simulink model "myStateFlow"  (R2018b)
settings: Solver=FixedStepAuto  StartTime=0.0  StopTime=2555  FixedStep=Ts  RelTol=1e-3
undefined symbols (not defined in the file or in its folder): DiscIntNeverNeededParam, plannedpath, pos0, posf
libraries: simulink x3
(part 1 of 2)
settings Model: Creator=sl  LastModifiedBy=sl

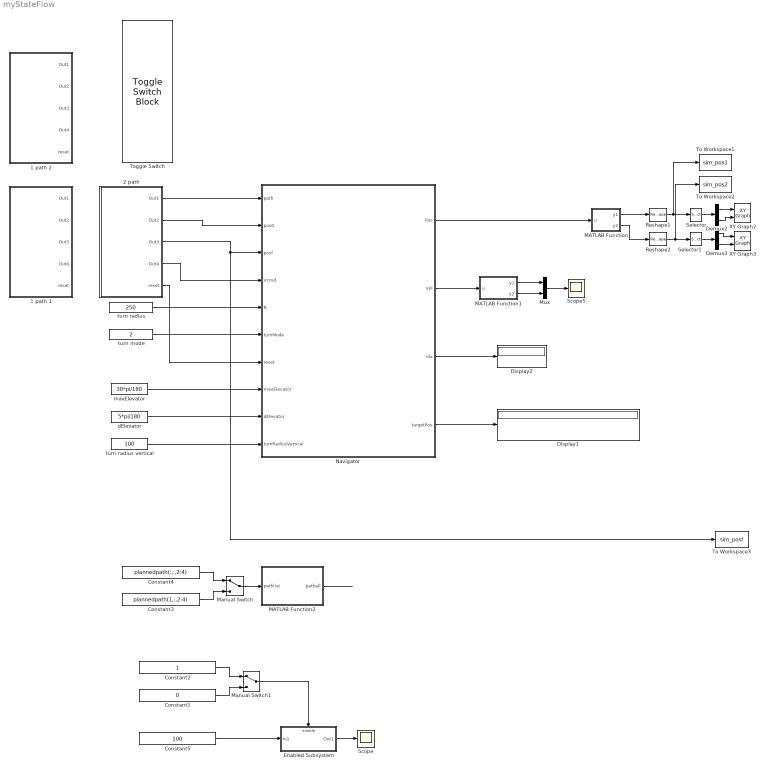
== system myStateFlow ==
  1 path 1 : Subsystem
  1 path 2 : Subsystem
  2 path : Subsystem
  Constant1 : Constant  Value=0  VectorParams1D=off
  Constant2 : Constant  VectorParams1D=off
  Constant3 : Constant  Value=plannedpath(1,:,2:4)  VectorParams1D=off
  Constant4 : Constant  Value=plannedpath(:,:,2:4)  VectorParams1D=off
  Constant5 : Constant  Value=100  VectorParams1D=off
  Demux2 : Demux  Outputs=2
  Demux3 : Demux  Outputs=2
  Display1 : Display
  Display2 : Display
  Enabled Subsystem : Subsystem  TreatAsAtomicUnit=on
  MATLAB Function : MATLAB Function  TreatAsAtomicUnit=on
  MATLAB Function1 : MATLAB Function  TreatAsAtomicUnit=on
  MATLAB Function2 : MATLAB Function  TreatAsAtomicUnit=on
  Manual Switch : ManualSwitch  varsize=on
  Manual Switch1 : ManualSwitch
  Mux : Mux  Inputs=2
  Navigator : Subsystem
  Reshape1 : Reshape
  Reshape2 : Reshape
  Scope : Scope
  Scope5 : Scope
  Selector : Selector  InputPortWidth=3  IndexOptions=Index vector (dialog)  Indices=[1 2]  OutputSizes=1
  Selector1 : Selector  InputPortWidth=3  IndexOptions=Index vector (dialog)  Indices=[1 2]  OutputSizes=1
  To Workspace1 : ToWorkspace  VariableName=sim_pos1  SaveFormat=Timeseries  SampleTime=-1
  To Workspace2 : ToWorkspace  VariableName=sim_pos2  SaveFormat=Timeseries  SampleTime=-1
  To Workspace3 : ToWorkspace  VariableName=sim_posf  SaveFormat=Timeseries  SampleTime=-1
  Toggle Switch : ToggleSwitchBlock  Tag=Reset  WebBlockId=267
      settings: Values={{'Off', 'On'}, [0 1]}
  XY Graph2 : simulink/Sinks/XY Graph  xmin=-2e4  xmax=2e4  ymin=-2e4  ymax=2e4  st=-1
  XY Graph3 : simulink/Sinks/XY Graph  xmin=-2e4  xmax=2e4  ymin=-2e4  ymax=2e4  st=-1
  dElevator : Constant  Value=5*pi/180
  maxElevator : Constant  Value=30*pi/180
  turn mode : Constant  Value=2  VectorParams1D=off
  turn radius : Constant  Value=250  VectorParams1D=off
  turn radius vertical : Constant  Value=100
  wires:
  Navigator/1(Pos) -> MATLAB Function/1(u)
  MATLAB Function/1(y1) -> Reshape1/1
  MATLAB Function/2(y2) -> Reshape2/1
  Demux2/1 -> XY Graph2/1
  Demux2/2 -> XY Graph2/2
  Demux3/2 -> XY Graph3/2
  Demux3/1 -> XY Graph3/1
  Reshape2/1 -> Selector1/1, To Workspace2/1
  Reshape1/1 -> To Workspace1/1, Selector/1
  Selector/1 -> Demux2/1
  Selector1/1 -> Demux3/1
  Navigator/2(Vel) -> MATLAB Function1/1(u)
  MATLAB Function1/1(y1) -> Mux/1
  MATLAB Function1/2(y2) -> Mux/2
  Mux/1 -> Scope5/1
  Navigator/3(idx) -> Display2/1
  Constant4/1 -> Manual Switch/1
  Constant3/1 -> Manual Switch/2
  Manual Switch/1 -> MATLAB Function2/1(pathlist)
  MATLAB Function2/1(pathall) -> ?
  2 path/3(Out3) -> Navigator/3(posf), To Workspace3/1
  2 path/1(Out1) -> Navigator/1(path)
  2 path/2(Out2) -> Navigator/2(pos0)
  2 path/4(Out4) -> Navigator/4(Vcmd)
  turn radius/1 -> Navigator/5(R)
  turn mode/1 -> Navigator/6(turnMode)
  maxElevator/1 -> Navigator/8(maxElevator)
  dElevator/1 -> Navigator/9(dElevator)
  turn radius vertical/1 -> Navigator/10("turnRadiusVertical ")
  Navigator/4(targetPos) -> Display1/1
  2 path/5(reset) -> Navigator/7(reset)
  Constant1/1 -> Manual Switch1/2
  Constant2/1 -> Manual Switch1/1
  Manual Switch1/1 -> Enabled Subsystem/Enable
  Constant5/1 -> Enabled Subsystem/1(In1)
  Enabled Subsystem/1(Out1) -> Scope/1

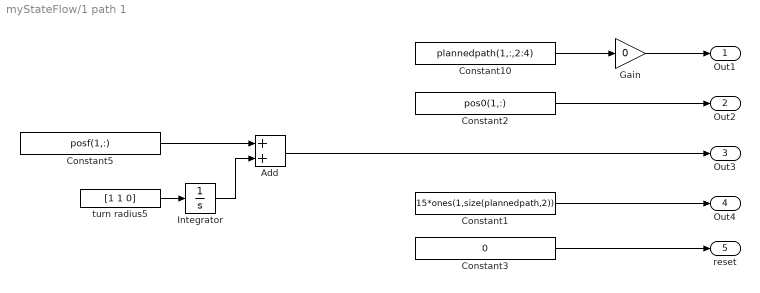
== system myStateFlow/1 path 1 ==
  Add : Sum
  Constant1 : Constant  Value=15*ones(1,size(plannedpath,2))  VectorParams1D=off
  Constant10 : Constant  Value=plannedpath(1,:,2:4)  VectorParams1D=off
  Constant2 : Constant  Value=pos0(1,:)  VectorParams1D=off
  Constant3 : Constant  Value=0  VectorParams1D=off
  Constant5 : Constant  Value=posf(1,:)  VectorParams1D=off
  Gain : Gain  Gain=0
  Integrator : Integrator
  turn radius5 : Constant  Value=[1 1 0]  VectorParams1D=off
  Out1 : Outport
  Out2 : Outport  Port=2
  Out3 : Outport  Port=3
  Out4 : Outport  Port=4
  reset : Outport  Port=5
  wires:
  Constant5/1 -> Add/1
  Add/1 -> Out3/1
  Integrator/1 -> Add/2
  Constant1/1 -> Out4/1
  turn radius5/1 -> Integrator/1
  Constant10/1 -> Gain/1
  Constant2/1 -> Out2/1
  Gain/1 -> Out1/1
  Constant3/1 -> reset/1

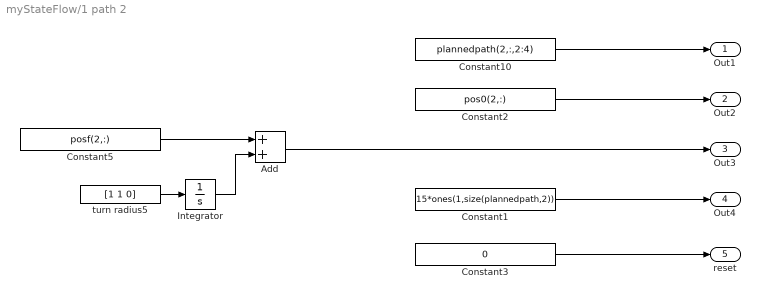
== system myStateFlow/1 path 2 ==
  Add : Sum
  Constant1 : Constant  Value=15*ones(1,size(plannedpath,2))  VectorParams1D=off
  Constant10 : Constant  Value=plannedpath(2,:,2:4)  VectorParams1D=off
  Constant2 : Constant  Value=pos0(2,:)  VectorParams1D=off
  Constant3 : Constant  Value=0  VectorParams1D=off
  Constant5 : Constant  Value=posf(2,:)  VectorParams1D=off
  Integrator : Integrator
  turn radius5 : Constant  Value=[1 1 0]  VectorParams1D=off
  Out1 : Outport
  Out2 : Outport  Port=2
  Out3 : Outport  Port=3
  Out4 : Outport  Port=4
  reset : Outport  Port=5
  wires:
  Constant2/1 -> Out2/1
  Constant10/1 -> Out1/1
  turn radius5/1 -> Integrator/1
  Constant1/1 -> Out4/1
  Integrator/1 -> Add/2
  Add/1 -> Out3/1
  Constant5/1 -> Add/1
  Constant3/1 -> reset/1

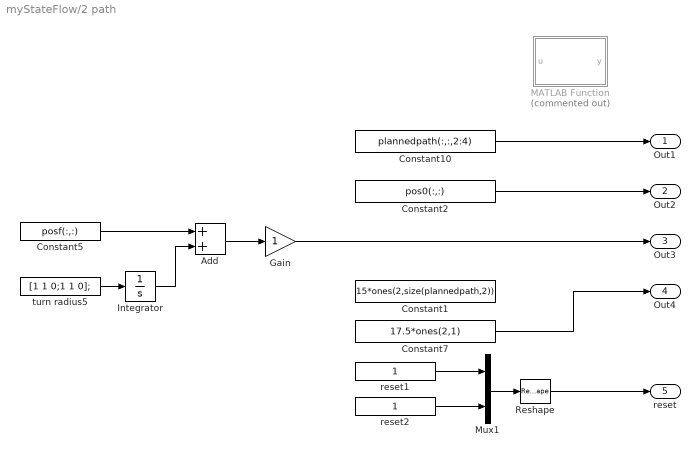
== system myStateFlow/2 path ==
  Add : Sum
  Constant1 : Constant  Value=15*ones(2,size(plannedpath,2))  VectorParams1D=off
  Constant10 : Constant  Value=plannedpath(:,:,2:4)  VectorParams1D=off
  Constant2 : Constant  Value=pos0(:,:)  VectorParams1D=off
  Constant5 : Constant  Value=posf(:,:)  VectorParams1D=off
  Constant7 : Constant  Value=17.5*ones(2,1)  VectorParams1D=off
  Gain : Gain
  Integrator : Integrator
  MATLAB Function : MATLAB Function  Commented=on  TreatAsAtomicUnit=on
  Mux1 : Mux  Inputs=2
  Reshape : Reshape  OutputDimensionality=Column vector (2-D)
  reset1 : Constant  VectorParams1D=off
  reset2 : Constant  VectorParams1D=off
  turn radius5 : Constant  Value=[1 1 0;1 1 0];  VectorParams1D=off
  Out1 : Outport
  Out2 : Outport  Port=2
  Out3 : Outport  Port=3
  Out4 : Outport  Port=4
  reset : Outport  Port=5
  wires:
  Constant2/1 -> Out2/1
  turn radius5/1 -> Integrator/1
  Integrator/1 -> Add/2
  Add/1 -> Gain/1
  Constant5/1 -> Add/1
  Constant7/1 -> Out4/1
  Gain/1 -> Out3/1
  Constant10/1 -> Out1/1
  Reshape/1 -> reset/1
  Mux1/1 -> Reshape/1
  reset1/1 -> Mux1/1
  reset2/1 -> Mux1/2

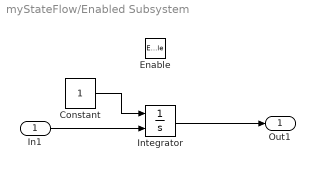
== system myStateFlow/Enabled Subsystem ==
  In1 : Inport
  Enable : EnablePort
  Constant : Constant
  Integrator : Integrator  InitialConditionSource=external
  Out1 : Outport
  wires:
  In1/1 -> Integrator/2
  Integrator/1 -> Out1/1
  Constant/1 -> Integrator/1

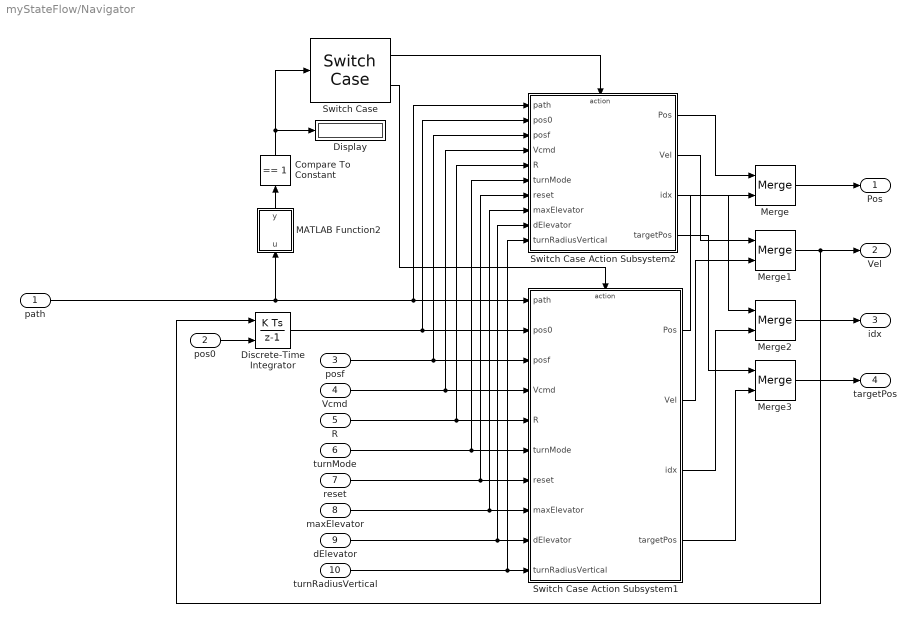
== system myStateFlow/Navigator ==
  path : Inport
  pos0 : Inport  Port=2
  posf : Inport  Port=3
  Vcmd : Inport  Port=4
  R : Inport  Port=5
  turnMode : Inport  Port=6
  reset : Inport  Port=7
  maxElevator : Inport  Port=8
  dElevator : Inport  Port=9
  "turnRadiusVertical " : Inport  Port=10
  Compare To Constant : simulink/Logic and Bit Operations/Compare To Constant  relop===  const=1  OutDataTypeStr=uint8
  Discrete-Time Integrator : DiscreteIntegrator  InitialConditionSource=external  SampleTime=-1  ICPrevOutput=DiscIntNeverNeededParam  ICPrevScaledInput=DiscIntNeverNeededParam
  Display : Display
  MATLAB Function2 : MATLAB Function  TreatAsAtomicUnit=on
  Merge{,1..3} (4 alike) : Merge
  Switch Case : SwitchCase
  Switch Case Action Subsystem1 : Subsystem  TreatAsAtomicUnit=on
  Switch Case Action Subsystem2 : Subsystem  TreatAsAtomicUnit=on
  Pos : Outport
  Vel : Outport  Port=2
  idx : Outport  Port=3
  targetPos : Outport  Port=4
  wires:
  pos0/1 -> Discrete-Time Integrator/2
  Switch Case Action Subsystem2/4(targetPos) -> Merge3/1
  Switch Case Action Subsystem1/4(targetPos) -> Merge3/2
  Merge3/1 -> targetPos/1
  "turnRadiusVertical "/1 -> Switch Case Action Subsystem1/10("turnRadiusVertical "), Switch Case Action Subsystem2/10("turnRadiusVertical ")
  dElevator/1 -> Switch Case Action Subsystem1/9(dElevator), Switch Case Action Subsystem2/9(dElevator)
  maxElevator/1 -> Switch Case Action Subsystem1/8(maxElevator), Switch Case Action Subsystem2/8(maxElevator)
  path/1 -> MATLAB Function2/1(u), Switch Case Action Subsystem1/1(path), Switch Case Action Subsystem2/1(path)
  reset/1 -> Switch Case Action Subsystem1/7(reset), Switch Case Action Subsystem2/7(reset)
  turnMode/1 -> Switch Case Action Subsystem1/6(turnMode), Switch Case Action Subsystem2/6(turnMode)
  Switch Case Action Subsystem2/2(Vel) -> Merge1/1
  Switch Case Action Subsystem2/1(Pos) -> Merge/1
  Switch Case Action Subsystem1/2(Vel) -> Merge1/2
  Switch Case Action Subsystem2/3(idx) -> Merge2/1
  Switch Case/2 -> Switch Case Action Subsystem1/Action
  Switch Case/1 -> Switch Case Action Subsystem2/Action
  posf/1 -> Switch Case Action Subsystem1/3(posf), Switch Case Action Subsystem2/3(posf)
  Merge1/1 -> Vel/1, Discrete-Time Integrator/1
  Merge2/1 -> idx/1
  Vcmd/1 -> Switch Case Action Subsystem1/4(Vcmd), Switch Case Action Subsystem2/4(Vcmd)
  MATLAB Function2/1(y) -> Compare To Constant/1
  R/1 -> Switch Case Action Subsystem1/5(R), Switch Case Action Subsystem2/5(R)
  Compare To Constant/1 -> Switch Case/1, Display/1
  Discrete-Time Integrator/1 -> Switch Case Action Subsystem1/2(pos0), Switch Case Action Subsystem2/2(pos0)
  Switch Case Action Subsystem1/3(idx) -> Merge2/2
  Switch Case Action Subsystem1/1(Pos) -> Merge/2
  Merge/1 -> Pos/1

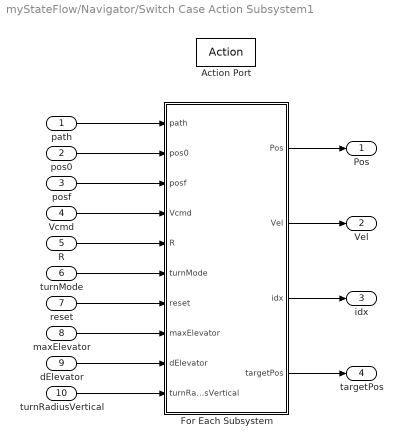
== system myStateFlow/Navigator/Switch Case Action Subsystem1 ==
  path : Inport
  pos0 : Inport  Port=2
  posf : Inport  Port=3
  Vcmd : Inport  Port=4
  R : Inport  Port=5
  turnMode : Inport  Port=6
  reset : Inport  Port=7
  maxElevator : Inport  Port=8
  dElevator : Inport  Port=9
  "turnRadiusVertical " : Inport  Port=10
  Action Port : ActionPort
  For Each Subsystem : Subsystem  TreatAsAtomicUnit=on
  Pos : Outport
  Vel : Outport  Port=2
  idx : Outport  Port=3
  targetPos : Outport  Port=4
  wires:
  For Each Subsystem/4(targetPos) -> targetPos/1
  "turnRadiusVertical "/1 -> For Each Subsystem/10("turnRadiusVertical ")
  dElevator/1 -> For Each Subsystem/9(dElevator)
  maxElevator/1 -> For Each Subsystem/8(maxElevator)
  reset/1 -> For Each Subsystem/7(reset)
  turnMode/1 -> For Each Subsystem/6(turnMode)
  path/1 -> For Each Subsystem/1(path)
  pos0/1 -> For Each Subsystem/2(pos0)
  posf/1 -> For Each Subsystem/3(posf)
  Vcmd/1 -> For Each Subsystem/4(Vcmd)
  R/1 -> For Each Subsystem/5(R)
  For Each Subsystem/1(Pos) -> Pos/1
  For Each Subsystem/2(Vel) -> Vel/1
  For Each Subsystem/3(idx) -> idx/1

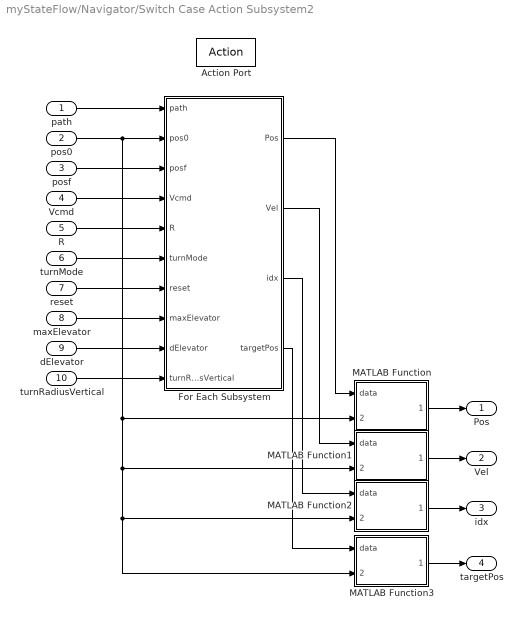
== system myStateFlow/Navigator/Switch Case Action Subsystem2 ==
  path : Inport
  pos0 : Inport  Port=2
  posf : Inport  Port=3
  Vcmd : Inport  Port=4
  R : Inport  Port=5
  turnMode : Inport  Port=6
  reset : Inport  Port=7
  maxElevator : Inport  Port=8
  dElevator : Inport  Port=9
  "turnRadiusVertical " : Inport  Port=10
  Action Port : ActionPort
  For Each Subsystem : Subsystem  TreatAsAtomicUnit=on
  MATLAB Function : MATLAB Function  TreatAsAtomicUnit=on
  MATLAB Function1 : MATLAB Function  TreatAsAtomicUnit=on
  MATLAB Function2 : MATLAB Function  TreatAsAtomicUnit=on
  MATLAB Function3 : MATLAB Function  TreatAsAtomicUnit=on
  Pos : Outport
  Vel : Outport  Port=2
  idx : Outport  Port=3
  targetPos : Outport  Port=4
  wires:
  MATLAB Function3/1(dataout) -> targetPos/1
  For Each Subsystem/4(targetPos) -> MATLAB Function3/1(data)
  "turnRadiusVertical "/1 -> For Each Subsystem/10("turnRadiusVertical ")
  dElevator/1 -> For Each Subsystem/9(dElevator)
  maxElevator/1 -> For Each Subsystem/8(maxElevator)
  reset/1 -> For Each Subsystem/7(reset)
  turnMode/1 -> For Each Subsystem/6(turnMode)
  MATLAB Function2/1(dataout) -> idx/1
  MATLAB Function1/1(dataout) -> Vel/1
  MATLAB Function/1(dataout) -> Pos/1
  For Each Subsystem/3(idx) -> MATLAB Function2/1(data)
  For Each Subsystem/2(Vel) -> MATLAB Function1/1(data)
  For Each Subsystem/1(Pos) -> MATLAB Function/1(data)
  R/1 -> For Each Subsystem/5(R)
  Vcmd/1 -> For Each Subsystem/4(Vcmd)
  posf/1 -> For Each Subsystem/3(posf)
  pos0/1 -> For Each Subsystem/2(pos0), MATLAB Function1/2(sizedata), MATLAB Function2/2(sizedata), MATLAB Function3/2(sizedata), MATLAB Function/2(sizedata)
  path/1 -> For Each Subsystem/1(path)

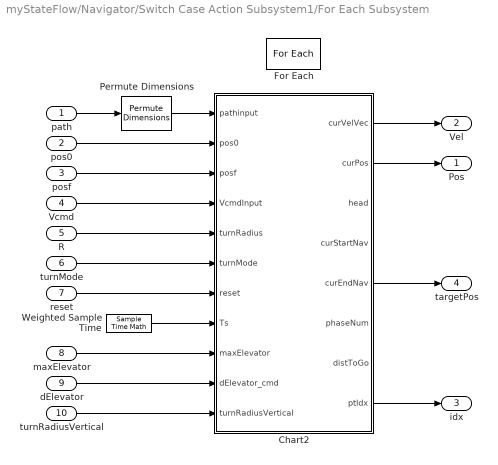
== system myStateFlow/Navigator/Switch Case Action Subsystem1/For Each Subsystem ==
  path : Inport  Partition=on  PartitionDimension=1  PartitionWidth=1  PartitionOffset=0
  pos0 : Inport  Port=2  Partition=on  PartitionDimension=1  PartitionWidth=1  PartitionOffset=0
  posf : Inport  Port=3  Partition=on  PartitionDimension=1  PartitionWidth=1  PartitionOffset=0
  Vcmd : Inport  Port=4  Partition=on  PartitionDimension=1  PartitionWidth=1  PartitionOffset=0
  R : Inport  Port=5
  turnMode : Inport  Port=6
  reset : Inport  Port=7  Partition=on  PartitionDimension=1  PartitionWidth=1  PartitionOffset=0
  maxElevator : Inport  Port=8
  dElevator : Inport  Port=9
  "turnRadiusVertical " : Inport  Port=10
  Chart2 : Stateflow chart  TreatAsAtomicUnit=on
  For Each : ForEach  DisableCoverage=on  IndexMode=One-based
  Permute Dimensions : PermuteDimensions  Order=[2,3,1]
  Weighted Sample Time : SampleTimeMath  TsampMathOp=Ts Only
  Pos : Outport  ConcatenationDimension=1
  Vel : Outport  Port=2  ConcatenationDimension=1
  idx : Outport  Port=3  ConcatenationDimension=1
  targetPos : Outport  Port=4  ConcatenationDimension=1
  wires:
  Chart2/5(curEndNav) -> targetPos/1
  turnMode/1 -> Chart2/6(turnMode)
  Chart2/8(ptIdx) -> idx/1
  "turnRadiusVertical "/1 -> Chart2/11(turnRadiusVertical)
  dElevator/1 -> Chart2/10(dElevator_cmd)
  maxElevator/1 -> Chart2/9(maxElevator)
  Weighted Sample Time/1 -> Chart2/8(Ts)
  reset/1 -> Chart2/7(reset)
  Chart2/2(curPos) -> Pos/1
  R/1 -> Chart2/5(turnRadius)
  Chart2/1(curVelVec) -> Vel/1
  Vcmd/1 -> Chart2/4(VcmdInput)
  pos0/1 -> Chart2/2(pos0)
  posf/1 -> Chart2/3(posf)
  path/1 -> Permute Dimensions/1
  Permute Dimensions/1 -> Chart2/1(pathinput)

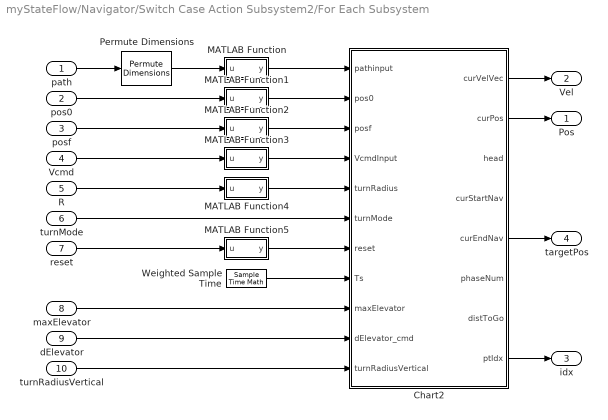
== system myStateFlow/Navigator/Switch Case Action Subsystem2/For Each Subsystem ==
  path : Inport
  pos0 : Inport  Port=2
  posf : Inport  Port=3
  Vcmd : Inport  Port=4
  R : Inport  Port=5
  turnMode : Inport  Port=6
  reset : Inport  Port=7
  maxElevator : Inport  Port=8
  dElevator : Inport  Port=9
  "turnRadiusVertical " : Inport  Port=10
  Chart2 : Stateflow chart  TreatAsAtomicUnit=on
  MATLAB Function : MATLAB Function  TreatAsAtomicUnit=on
  MATLAB Function1 : MATLAB Function  TreatAsAtomicUnit=on
  MATLAB Function2 : MATLAB Function  TreatAsAtomicUnit=on
  MATLAB Function3 : MATLAB Function  TreatAsAtomicUnit=on
  MATLAB Function4 : MATLAB Function  TreatAsAtomicUnit=on
  MATLAB Function5 : MATLAB Function  TreatAsAtomicUnit=on
  Permute Dimensions : PermuteDimensions  Order=[2,3,1]
  Weighted Sample Time : SampleTimeMath  TsampMathOp=Ts Only
  Pos : Outport
  Vel : Outport  Port=2
  idx : Outport  Port=3
  targetPos : Outport  Port=4
  wires:
  MATLAB Function5/1(y) -> Chart2/7(reset)
  Chart2/5(curEndNav) -> targetPos/1
  "turnRadiusVertical "/1 -> Chart2/11(turnRadiusVertical)
  dElevator/1 -> Chart2/10(dElevator_cmd)
  maxElevator/1 -> Chart2/9(maxElevator)
  reset/1 -> MATLAB Function5/1(u)
  turnMode/1 -> Chart2/6(turnMode)
  MATLAB Function4/1(y) -> Chart2/5(turnRadius)
  MATLAB Function3/1(y) -> Chart2/4(VcmdInput)
  MATLAB Function2/1(y) -> Chart2/3(posf)
  MATLAB Function1/1(y) -> Chart2/2(pos0)
  MATLAB Function/1(y) -> Chart2/1(pathinput)
  Permute Dimensions/1 -> MATLAB Function/1(u)
  path/1 -> Permute Dimensions/1
  posf/1 -> MATLAB Function2/1(u)
  pos0/1 -> MATLAB Function1/1(u)
  Vcmd/1 -> MATLAB Function3/1(u)
  Chart2/8(ptIdx) -> idx/1
  Chart2/1(curVelVec) -> Vel/1
  R/1 -> MATLAB Function4/1(u)
  Weighted Sample Time/1 -> Chart2/8(Ts)
  Chart2/2(curPos) -> Pos/1

== matlab function myStateFlow/MATLAB Function ==
  data: u input; y1 output; y2 output
function [y1,y2]= fcn(u)

y1 = u(1,:);
y2 = u(2,:);

== matlab function myStateFlow/MATLAB Function1 ==
  data: u input; y1 output; y2 output
function [y1,y2]= fcn(u)

y1 = norm(u(1,:));
y2 = norm(u(1,:));

== matlab function myStateFlow/MATLAB Function2 ==
  data: pathlist input; pathall output
function pathall = formPathList(pathlist)
% 将变长度航路转换为固定长度航路，便于后续处理
maxPathNum = 10;
maxPathPointNum = 100;
pathall = zeros(maxPathNum,maxPathPointNum,3);
[realPathNum,realPtNum,~] = size(pathlist);
if realPathNum>maxPathNum || realPtNum>maxPathPointNum
    error('The dimensions of pathlist exceed limits') ;
end
for i_path = 1:realPathNum
    pathall(i_path,1:realPtNum,:) = pathlist(i_path,:,:);
end

== matlab function myStateFlow/2 path/MATLAB Function ==
  data: u input; y output
function y = fcn(u)
u(2,:,:) = zeros(size(u(2,:,:)));
y = u;

== matlab function myStateFlow/Navigator/MATLAB Function2 ==
  data: u input; y output
function y = fcn(u)
if size(u,1) == 1
    y = 1;
else
    y = 0;
end

== stateflow chart myStateFlow/Navigator/Switch Case Action Subsystem1/For Each Subsystem/Chart2 ==
  state InitialPhase
    % turnMode 转弯模式 1折现转弯 2圆弧切线转弯
    en:
    ptIdx = 1;  % 当前阶段起始点在path点集中的序号
    % 导航点的位置向量
    [path,path_h,path_v] = calValidNavPts(pos0,pathinput,posf);
    Vcmd = [VcmdInput(1),VcmdInput];
    % 导航点的时间向量
    numPts = size(path,1);%determineNumPts; % 导航点数
    curPos = path(1,:); % 初始导航点作为当前阶段的目标
    phaseNum = 1;
    turnInPos = zeros(1,3);
    turnOutPos = zeros(1,3);
    curStartNav = zeros(1,3);
    curEndNav = zeros(1,3);
    curVelVec = zeros(1,3);
    curVel = zeros(1);
    posErr = zeros(1);
  state Hover
    en:
    head = 0;
    curPos = pos0;
    curVel = Vcmd(1);
    du:
    head = head+0.1*Ts;
    curVelVec = ([cos(head) sin(head) 0;-sin(head) cos(head) 0;0 0 1]*[curVel;0;0])';
    curPos = curPos + curVelVec*Ts;
    curStartNav = [0 0 0];
    curEndNav = [0 0 0];
    phaseNum = -1;
    distToGo = -1;
    ptIdx = -1;
  state MainLoop
    state linePhase
      % ------------------------------------------------------------------------------------------------
      en:
      while 1 % 跳过连续的重复点
      curStartNav = path(ptIdx,1:3);  % 当前导航段的起始点位置
      curEndNav = path(ptIdx+1,1:3); % 当前导航段的终点位置
      curVel = Vcmd(min(ptIdx,length(Vcmd))); % 当前导航段的速度
      if isequal(curStartNav(1:2),curEndNav(1:2)) % 判断连续的两个导航点是否重合
      if ptIdx>=numPts-1
      send(event_arriveEnd)
      break
      end
      ptIdx = ptIdx+1;
      else
      break
      end
      end
      % 当前导航段速度矢量
      curVelVec = curVel*(curEndNav-curPos)/(norm(curEndNav-curPos)+eps);
      head = atan2(curVelVec(2),curVelVec(1));
      elevator = rem(atan2(curVelVec(3),norm(curVelVec(1:2))),pi);
      posErr = 0.001;%max(Ts*curVel,0.01); % 用于判断是否到达的误差
      height0 = curPos(3);
      % 计算转弯切入点turnInPos和切出点位置turnOutPos
      [turnInPos,turnOutPos] = calTurnInOutPos();
      % ------------------------------------------------------------------------------------------------
      du:
      path = calValidNavPts(pos0,pathinput,posf);
      elevator = calElevatorForHeightManuv();
      curVelVec = rotateVelVec();
      curPos = curPos + curVelVec*Ts;
      [distToGo,skipTurnFlag] = determineArriveEvent();
      phaseNum = 2;
    state turnPhase
      en:
      path = calValidNavPts(pos0,pathinput,posf);
      [turnHeadVel,turnElvVel,headToTurn,elevatorToTurn]...
      = calTurnPos();
      head = atan2(curVelVec(2),curVelVec(1));
      elevator = rem(atan2(curVelVec(3),curVelVec(2)),pi);
      head0 = head;
      elevator0 = elevator;
      flagHeadComplete = 0;
      flagElvComplete = 1; % 转弯时不考虑高度机动
      TESTFUNC()
      du:
      % TODO
      path = calValidNavPts(pos0,pathinput,posf);
      head = head + turnHeadVel*Ts;
      elevator = elevator + turnElvVel*Ts;
      if abs(head-head0)>=headToTurn
      head = head0+headToTurn;
      turnHeadVel = 0;
      flagHeadComplete = 1;
      end
      if abs(elevator-elevator0)>=elevatorToTurn
      elevator = elevator0+elevatorToTurn;
      turnElvVel = 0;
      flagElvComplete = 1;
      end
      if flagHeadComplete == 1 && flagElvComplete ==1
      send(event_turnComplete)
      end
      curVelVec = updateVelForTurn();
      curPos = curPos + curVelVec*Ts;
      TESTFUNC()
    state EndPhase
      en:
      du:
      path = calValidNavPts(pos0,pathinput,posf);
      [curVelVec,head] = updateVelForEndphase();
      curPos = curPos + curVelVec*Ts;
      phaseNum = 3;
    turnPhase -> linePhase : event_turnComplete
        | {ptIdx = ptIdx+1;}
    (junction 52) -> linePhase [order 1] : [turnMode==1||skipTurnFlag<0]
        | {ptIdx = ptIdx+1;}
    (junction 52) -> turnPhase [order 2] : [turnMode==2&&skipTurnFlag>=0]
    linePhase -> (junction 17) : [event_arrive||event_arriveEnd]
    (junction 17) -> (junction 52) [order 2] : [ptIdx<numPts-1]
    (junction 17) -> EndPhase [order 1] : [ptIdx>=numPts-1||event_arriveEnd]
  (default) -> InitialPhase
  InitialPhase -> Hover [order 2] : [sum(sum(sum(abs(pathinput))))<eps]
  MainLoop -> InitialPhase : [hasChanged(reset)]
  InitialPhase -> linePhase [order 1] : [sum(sum(sum(abs(pathinput))))>=eps]
  data: numPts_ function_output; curVelVec_ function_output; dhead function_output; velVec function_output; out function_output; skipFlag function_output; curVelVec_ function_output; inPos function_output; outPos function_output; path_ function_output; path_h_ function_output; initialpos function_input; pathlist function_input; finalpos function_input; path_v_ function_output; elevator_ function_output; turnAngleVel_h function_output; turnAngleVel_e function_output; angleToTurn_h function_output; angleToTurn_e function_output; pathinput input; pos0 input; posf input; VcmdInput input; numPts local; endTime local; curVel local size=1; posDim local; path local; timeSeq local; turnRadius input; turnInPos local; turnOutPos local; curVelVec output; curPos output; posErr local; tempCurVelVec local; head output; curStartNav output; curEndNav output; phaseNum output; distToGo output; ptIdx output; turnAngleVel local; headToTurn local; elevatorToTurn local; turnElvVel local; turnHeadVel local; elevator local; flagHeadComplete local; flagElvComplete local; head0 local; elevator0 local; Vcmd local; turnMode input size=1; reset input; Ts input; dElevator local; path_h local; path_v local; height0 local; maxElevator input; dElevator_cmd input; turnRadiusVertical input; skipTurnFlag local
  events: event_arrive local FUNCTION_CALL_EVENT; event_arriveEnd local FUNCTION_CALL_EVENT; event_turnComplete local FUNCTION_CALL_EVENT; event_goToEnd local FUNCTION_CALL_EVENT; event_skip local FUNCTION_CALL_EVENT
  function numPts_ = determineNumPts:
    | function numPts_ = determineNumPts
    | nRow = size(path,1); % 导航点数
    | numPts_ = nRow;
    | for i = nRow:-1:2
    |     if ~isequal(path(i,:),path(i-1,:))
    |         numPts_ = i; 
    |         break;
    |     end
    | end
    | test = 1;
  function [curVelVec_,dhead] = updateVelForEndphase:
    | function [curVelVec_,dhead] = updateVelForEndphase
    | % head_ = atan2(curVelVec(2),curVelVec(1));
    | dhead = 2*pi/180*Ts;
    | curVelVec_h = [curVelVec(1:2),0]';
    | tempCurVelVec = curVel*curVelVec_h/norm(curVelVec_h);
    | tempCurVelVec = [...
    |      cos(dhead) sin(dhead) 0;
    |     -sin(dhead) cos(dhead) 0;
    |               0          0 1;]*tempCurVelVec;
    | curVelVec_ = tempCurVelVec';
  function velVec = rotateVelVec:
    | function velVec = rotateVelVec
    | Mz = [cos(head) sin(head) 0;
    |      -sin(head) cos(head) 0;
    |               0         0 1;];
    | My = [cos(-elevator) 0 -sin(-elevator);
    |                   0 1              0;
    |       sin(-elevator) 0  cos(-elevator)];        
    | velVec = (My*Mz)'*[curVel;0;0];
    | velVec = velVec';
  function [out,skipFlag] = determineArriveEvent:
    | function [out,skipFlag] = determineArriveEvent
    | out = norm(curPos(1:2)-turnInPos(1:2));
    | % xflag = curPos(1)>=max([curStartNav(1),curEndNav(1)]) || ...
    | %         curPos(1)< min([curStartNav(1),curEndNav(1)]);
    | % yflag = curPos(2)>=max([curStartNav(2),curEndNav(2)]) || ...
    | %         curPos(2)< min([curStartNav(2),curEndNav(2)]);    
    | vec1 = turnInPos - curPos;
    | vec1(3) = 0;
    | vec1 = vec1/norm(vec1);
    | vec2 = turnInPos - curStartNav;
    | vec2(3) = 0;
    | vec2 = vec2/norm(vec2);
    | vec3 = curEndNav - curStartNav;
    | vec3(3) = 0;
    | vec3 = vec3/norm(vec3);
    | passFlag = dot([vec1],[vec2]);
    | skipFlag = dot([vec1],[vec3]);
    | if out<=posErr || passFlag<-1e-6
    | %     curPos(1:2) = turnInPos(1:2); % 将水平位置修正到期望位置，并保留当前高度
    |     send(event_arrive)
    | end
    | % if skipFlag<-1e-6
    | %     send(event_skip)
    | % end
  function curVelVec_ = updateVelForTurn:
    | function curVelVec_ = updateVelForTurn()
    | dhead = turnHeadVel*Ts;
    | delevator = turnElvVel*Ts;
    | curVelVec_h = [curVelVec(1:2),0]';
    | tempCurVelVec = curVel*curVelVec_h/norm(curVelVec_h);
    | M_h = [...
    |      cos(dhead) sin(dhead) 0;
    |     -sin(dhead) cos(dhead) 0;
    |               0          0 1;];
    | M_e = [...
    |      cos(delevator) 0 -sin(delevator);
    |      0             1              0;
    |      sin(delevator) 0  cos(delevator);];          
    | temp = (M_e*M_h)'*tempCurVelVec;
    | curVelVec_ = temp';
  function [inPos,outPos] =calTurnInOutPos:
    | function [inPos,outPos] =calTurnInOutPos
    | inPos = curEndNav;
    | outPos = curEndNav;
    | if turnMode == 1
    |     inPos = curEndNav;
    |     outPos = curEndNav;
    | elseif turnMode == 2
    |     if ptIdx == numPts-1 % 当处于最后一段航线时
    |         inPos = curEndNav;
    |         outPos = -999*ones(size(path(ptIdx+1,1:3)));
    |     else
    |         nextNav = path(ptIdx+2,1:3);
    |         curVec = curEndNav-curStartNav;
    |         curVec(3) = 0; % 不考虑高度
    |         nextVec = nextNav-curEndNav;
    |         nextVec(3) = 0;
    |         lengthCurLine = norm(curVec);
    |         lengthNextLine = norm(nextVec);
    |         if lengthNextLine ~= 0
    |             %             if lengthCurLine<=dist || lengthNextLine<=dist
    |             %                 R = 1/2*min([lengthCurLine,lengthNextLine,dist]);
    |             %                 %             error('Turn radius is larger than the length of some path, which may cause unexpected results!');
    |             %             else
    |             %                 R = turnRadius;
    |             %             end
    |             R = turnRadius;
    |             angle1 = acos(dot([nextVec]/lengthNextLine,[curVec]/lengthCurLine));%asin(sum(cross([nextVec]/lengthNextLine,[curVec]/lengthCurLine)));
    |             angle_half = angle1/2;
    |             dist = R/abs(tan(pi/2-abs(angle_half)));
    |             while 1
    |                 if lengthCurLine<=dist || lengthNextLine<=dist
    |                     dist = 0.95*min(lengthCurLine,lengthNextLine);
    |                 else
    |                     break
    |                 end
    |             end
    |             inPos = curEndNav-curVec*dist/norm(curVec);
    |             outPos = curEndNav+nextVec*dist/norm(nextVec);
    |         else
    |             inPos = curEndNav;
    |             outPos = curEndNav;
    |         end
    |         if isnan(outPos)
    |             sl = 1;
    |         end
    |     end
    | end
    | if 0 % TEST
    |     figure;
    |     plot(curPos(1),curPos(2),'k+');hold on;
    |     plot(curEndNav(1),curEndNav(2),'ro');hold on;
    |     plot(curStartNav(1),curStartNav(2),'ro');hold on;
    |     plot(inPos(1),inPos(2),'bo');hold on;
    |     plot(outPos(1),outPos(2),'bo');hold on;
    |     plot(nextNav(1),nextNav(2),'ro');hold on;
    |     plot([curStartNav(1) curEndNav(1) nextNav(1)],[curStartNav(2) curEndNav(2) nextNav(2)],'r');hold on;
    |     axis equal
    |     grid on;
    | end
    | test = 1;
  function TESTFUNC:
    | function TESTFUNC
    | coder.extrinsic('fprintf')
    | % fprintf('\n');
    | % fprintf('head: %.2f\n',head*57.3);
    | % fprintf('headTurned: %.2f\n', head*57.3-head0*57.3);
    | % fprintf('head_flag: %d\n', abs(head-head0)>=headToTurn);
    | % fprintf('elevator_flag: %d\n', abs(elevator-elevator0)>=elevatorToTurn);
    | % fprintf('ptIdx: %d\n',ptIdx);
    | if isnan(curVelVec)
    |     sl = 1;
    | end
    | if isnan(sum(curPos))
    |     sl = 1;
    | end
    | % if isnan(headToTurn)
    | %     sl = 1;
    | % end
    | if ptIdx >=30
    |     sl = 1;
    | end
  function [path_,path_h_,path_v_] = calValidNavPts(initialpos,pathlist,finalpos):
    | function [path_,path_h_,path_v_] = calValidNavPts(initialpos,pathlist,finalpos)
    | %% 计算包括当前位置和额外指定终点在内的完整航路
    | % initialpos：进入导航模式时的单位所在位置
    | % pathlist：航路点序列
    | % finalpos:终点位置
    | %% 计算过程
    | path_ = [initialpos(1:3);pathlist(:,1:3);finalpos(1:3)]; % 形成完整航路数组
    | % path_最小点数为4（1起点+2航路+1终点），航路规划算法给出的pathlist中，
    | % 由[0,0,0]填充末尾不存在的位置点，因此在实际导航时，需将这些点去掉
    | for i = size(path_,1)-1:-1:4 
    |     if norm(path_(i,:)) == 0 % 处理末尾的[0,0,0],填充为终点位置坐标
    |         path_(i,:) = finalpos(1:3);
    |     else
    |         break;
    |     end
    | end
    | path_h_ = [path_(:,1:2) 0*path_(:,3)];
    | path_v_ = [0*path_(:,1) 0*path_(:,2) path_(:,3)];
    | test = 1; % 用于加断点的行
  function elevator_ = calElevatorForHeightManuv:
    | function elevator_ = calElevatorForHeightManuv
    | elevatorCmd = maxElevator;
    | dElevatorCmd = dElevator_cmd;
    | turnR = turnRadiusVertical;
    | premeter = 2*pi*turnR;
    | arcLength = premeter*2*elevatorCmd/2/pi;
    | tSpend = arcLength/curVel;
    | dist = turnR*tan(elevatorCmd);
    | turnH = dist*sin(elevatorCmd); 
    | 
    | targetHeight = path(ptIdx+1,3);
    | % startHeight = path(ptIdx,3);
    | startHeight = height0;
    | currentHeight = curPos(3);
    | restHeight = targetHeight-currentHeight;
    | passedHeight = currentHeight-startHeight;
    | absoluteErrHeight = targetHeight-startHeight;
    | if abs(absoluteErrHeight)>2*turnH 
    |     if elevator<=elevatorCmd && abs(passedHeight)<=turnH
    |         dElevator_ = sign(absoluteErrHeight)*dElevatorCmd;
    |         phase = 1;
    |     elseif abs(passedHeight)>abs(absoluteErrHeight)-turnH 
    |         dElevator_ = -sign(absoluteErrHeight)*dElevatorCmd;
    |         phase = 3;
    |     else
    |         dElevator_ = 0;
    |         phase = 2;
    |     end
    | else
    |     if abs(passedHeight)<1/2*abs(absoluteErrHeight)
    |         dElevator_ = sign(absoluteErrHeight)*dElevatorCmd;
    |         phase = 1;
    |     else
    |         dElevator_ = -sign(absoluteErrHeight)*dElevatorCmd;
    |         phase = 3;
    |     end
    | end
    | switch phase
    |     case 1
    |         elevator_ = elevator + dElevator_*Ts;
    |         if absoluteErrHeight>0
    |             elevator_ = min(elevator_,elevatorCmd);
    |         else
    |             elevator_ = max(elevator_,-elevatorCmd);
    |         end
    |     case 2
    |         elevator_ = sign(absoluteErrHeight)*elevatorCmd;
    |     case 3
    |         elevator_ = elevator + dElevator_*Ts;
    |         if absoluteErrHeight>0
    |             elevator_ = max(elevator_,0);
    |         else
    |             elevator_ = min(elevator_,0);
    |         end        
    |     otherwise
    |         elevator_ = 0;
    | end
  function [turnAngleVel_h,turnAngleVel_e,angleToTurn_h,angleToTurn_e] ...:
    | function [turnAngleVel_h,turnAngleVel_e,angleToTurn_h,angleToTurn_e] ...
    |     = calTurnPos()
    | nextNav = path(ptIdx+2,1:3);
    | curVec = curEndNav-curStartNav;
    | % curVec = curEndNav-curPos; 
    | curVec(3) = 0;
    | nextVec = nextNav-curEndNav;
    | nextVec(3) = 0;
    | lengthCurLine = norm(curVec);
    | lengthNextLine = norm(nextVec);
    | if lengthNextLine ~= 0 && lengthCurLine ~= 0
    |     angleToTurn_h_sym = asin(sum(cross(nextVec/lengthNextLine,curVec/lengthCurLine)));
    |     angleToTurn_h = acos(sum(dot(nextVec/lengthNextLine,curVec/lengthCurLine)));
    | else
    |     angleToTurn_h_sym = 0;
    |     angleToTurn_h = 0;
    | end
    | curElv = rem(atan2(curVec(3),curVec(2)),pi);
    | nextElv = rem(atan2(nextVec(3),nextVec(2)),pi);
    | if angleToTurn_h_sym >= 0
    |     flag_h = -1;  
    | else
    |     flag_h = 1;
    | end
    | perimeter = 2*pi*turnRadius;
    | timePerCircle = perimeter/curVel;
    | turnAngleVel_h = flag_h*2*pi/timePerCircle;%abs(angleToTurn_h)/timePerCircle;
    | turnAngleVel_e = (nextElv-curElv)/timePerCircle;
    | angleToTurn_h = abs(angleToTurn_h);
    | angleToTurn_e = nextElv-curElv;
    | if isnan(angleToTurn_h)
    |     sl = 1;
    | end

== stateflow chart myStateFlow/Navigator/Switch Case Action Subsystem2/For Each Subsystem/Chart2 ==
  state InitialPhase
    % turnMode 转弯模式 1折现转弯 2圆弧切线转弯
    en:
    ptIdx = 1;  % 当前阶段起始点在path点集中的序号
    % 导航点的位置向量
    [path,path_h,path_v] = calValidNavPts(pos0,pathinput,posf);
    Vcmd = [VcmdInput(1),VcmdInput];
    % 导航点的时间向量
    numPts = size(path,1);%determineNumPts; % 导航点数
    curPos = path(1,:); % 初始导航点作为当前阶段的目标
    phaseNum = 1;
    turnInPos = zeros(1,3);
    turnOutPos = zeros(1,3);
    curStartNav = zeros(1,3);
    curEndNav = zeros(1,3);
    curVelVec = zeros(1,3);
    curVel = zeros(1);
    posErr = zeros(1);
  state Hover
    en:
    head = 0;
    curPos = pos0;
    curVel = Vcmd(1);
    du:
    head = head+0.1*Ts;
    curVelVec = ([cos(head) sin(head) 0;-sin(head) cos(head) 0;0 0 1]*[curVel;0;0])';
    curPos = curPos + curVelVec*Ts;
    curStartNav = [0 0 0];
    curEndNav = [0 0 0];
    phaseNum = -1;
    distToGo = -1;
    ptIdx = -1;
  state MainLoop
    state linePhase
      % ------------------------------------------------------------------------------------------------
      en:
      while 1 % 跳过连续的重复点
      curStartNav = path(ptIdx,1:3);  % 当前导航段的起始点位置
      curEndNav = path(ptIdx+1,1:3); % 当前导航段的终点位置
      curVel = Vcmd(min(ptIdx,length(Vcmd))); % 当前导航段的速度
      if isequal(curStartNav(1:2),curEndNav(1:2)) % 判断连续的两个导航点是否重合
      if ptIdx>=numPts-1
      send(event_arriveEnd)
      break
      end
      ptIdx = ptIdx+1;
      else
      break
      end
      end
      % 当前导航段速度矢量
      curVelVec = curVel*(curEndNav-curPos)/(norm(curEndNav-curPos)+eps);
      head = atan2(curVelVec(2),curVelVec(1));
      elevator = rem(atan2(curVelVec(3),norm(curVelVec(1:2))),pi);
      posErr = 0.001;%max(Ts*curVel,0.01); % 用于判断是否到达的误差
      height0 = curPos(3);
      % 计算转弯切入点turnInPos和切出点位置turnOutPos
      [turnInPos,turnOutPos] = calTurnInOutPos();
      % ------------------------------------------------------------------------------------------------
      du:
      path = calValidNavPts(pos0,pathinput,posf);
      elevator = calElevatorForHeightManuv();
      curVelVec = rotateVelVec();
      curPos = curPos + curVelVec*Ts;
      [distToGo,skipTurnFlag] = determineArriveEvent();
      phaseNum = 2;
    state turnPhase
      en:
      path = calValidNavPts(pos0,pathinput,posf);
      [turnHeadVel,turnElvVel,headToTurn,elevatorToTurn]...
      = calTurnPos();
      head = atan2(curVelVec(2),curVelVec(1));
      elevator = rem(atan2(curVelVec(3),curVelVec(2)),pi);
      head0 = head;
      elevator0 = elevator;
      flagHeadComplete = 0;
      flagElvComplete = 1; % 转弯时不考虑高度机动
      TESTFUNC()
      du:
      % TODO
      path = calValidNavPts(pos0,pathinput,posf);
      head = head + turnHeadVel*Ts;
      elevator = elevator + turnElvVel*Ts;
      if abs(head-head0)>=headToTurn
      head = head0+headToTurn;
      turnHeadVel = 0;
      flagHeadComplete = 1;
      end
      if abs(elevator-elevator0)>=elevatorToTurn
      elevator = elevator0+elevatorToTurn;
      turnElvVel = 0;
      flagElvComplete = 1;
      end
      if flagHeadComplete == 1 && flagElvComplete ==1
      send(event_turnComplete)
      end
      curVelVec = updateVelForTurn();
      curPos = curPos + curVelVec*Ts;
      TESTFUNC()
    state EndPhase
      en:
      du:
      path = calValidNavPts(pos0,pathinput,posf);
      [curVelVec,head] = updateVelForEndphase();
      curPos = curPos + curVelVec*Ts;
      phaseNum = 3;
    turnPhase -> linePhase : event_turnComplete
        | {ptIdx = ptIdx+1;}
    (junction 52) -> linePhase [order 1] : [turnMode==1||skipTurnFlag<0]
        | {ptIdx = ptIdx+1;}
    (junction 52) -> turnPhase [order 2] : [turnMode==2&&skipTurnFlag>=0]
    linePhase -> (junction 17) : [event_arrive||event_arriveEnd]
    (junction 17) -> (junction 52) [order 2] : [ptIdx<numPts-1]
    (junction 17) -> EndPhase [order 1] : [ptIdx>=numPts-1||event_arriveEnd]
  (default) -> InitialPhase
  InitialPhase -> Hover [order 2] : [sum(sum(sum(abs(pathinput))))<eps]
  MainLoop -> InitialPhase : [hasChanged(reset)]
  InitialPhase -> linePhase [order 1] : [sum(sum(sum(abs(pathinput))))>=eps]
  data: numPts_ function_output; curVelVec_ function_output; dhead function_output; velVec function_output; out function_output; skipFlag function_output; curVelVec_ function_output; inPos function_output; outPos function_output; path_ function_output; path_h_ function_output; initialpos function_input; pathlist function_input; finalpos function_input; path_v_ function_output; elevator_ function_output; turnAngleVel_h function_output; turnAngleVel_e function_output; angleToTurn_h function_output; angleToTurn_e function_output; pathinput input; pos0 input; posf input; VcmdInput input; numPts local; endTime local; curVel local size=1; posDim local; path local; timeSeq local; turnRadius input; turnInPos local; turnOutPos local; curVelVec output; curPos output; posErr local; tempCurVelVec local; head output; curStartNav output; curEndNav output; phaseNum output; distToGo output; ptIdx output; turnAngleVel local; headToTurn local; elevatorToTurn local; turnElvVel local; turnHeadVel local; elevator local; flagHeadComplete local; flagElvComplete local; head0 local; elevator0 local; Vcmd local; turnMode input size=1; reset input; Ts input; dElevator local; path_h local; path_v local; height0 local; maxElevator input; dElevator_cmd input; turnRadiusVertical input; skipTurnFlag local
  events: event_arrive local FUNCTION_CALL_EVENT; event_arriveEnd local FUNCTION_CALL_EVENT; event_turnComplete local FUNCTION_CALL_EVENT; event_goToEnd local FUNCTION_CALL_EVENT; event_skip local FUNCTION_CALL_EVENT
  function numPts_ = determineNumPts:
    | function numPts_ = determineNumPts
    | nRow = size(path,1); % 导航点数
    | numPts_ = nRow;
    | for i = nRow:-1:2
    |     if ~isequal(path(i,:),path(i-1,:))
    |         numPts_ = i; 
    |         break;
    |     end
    | end
    | test = 1;
  function [curVelVec_,dhead] = updateVelForEndphase:
    | function [curVelVec_,dhead] = updateVelForEndphase
    | % head_ = atan2(curVelVec(2),curVelVec(1));
    | dhead = 2*pi/180*Ts;
    | curVelVec_h = [curVelVec(1:2),0]';
    | tempCurVelVec = curVel*curVelVec_h/norm(curVelVec_h);
    | tempCurVelVec = [...
    |      cos(dhead) sin(dhead) 0;
    |     -sin(dhead) cos(dhead) 0;
    |               0          0 1;]*tempCurVelVec;
    | curVelVec_ = tempCurVelVec';
  function velVec = rotateVelVec:
    | function velVec = rotateVelVec
    | Mz = [cos(head) sin(head) 0;
    |      -sin(head) cos(head) 0;
    |               0         0 1;];
    | My = [cos(-elevator) 0 -sin(-elevator);
    |                   0 1              0;
    |       sin(-elevator) 0  cos(-elevator)];        
    | velVec = (My*Mz)'*[curVel;0;0];
    | velVec = velVec';
  function [out,skipFlag] = determineArriveEvent:
    | function [out,skipFlag] = determineArriveEvent
    | out = norm(curPos(1:2)-turnInPos(1:2));
    | % xflag = curPos(1)>=max([curStartNav(1),curEndNav(1)]) || ...
    | %         curPos(1)< min([curStartNav(1),curEndNav(1)]);
    | % yflag = curPos(2)>=max([curStartNav(2),curEndNav(2)]) || ...
    | %         curPos(2)< min([curStartNav(2),curEndNav(2)]);    
    | vec1 = turnInPos - curPos;
    | vec1(3) = 0;
    | vec1 = vec1/norm(vec1);
    | vec2 = turnInPos - curStartNav;
    | vec2(3) = 0;
    | vec2 = vec2/norm(vec2);
    | vec3 = curEndNav - curStartNav;
    | vec3(3) = 0;
    | vec3 = vec3/norm(vec3);
    | passFlag = dot([vec1],[vec2]);
    | skipFlag = dot([vec1],[vec3]);
    | if out<=posErr || passFlag<-1e-6
    | %     curPos(1:2) = turnInPos(1:2); % 将水平位置修正到期望位置，并保留当前高度
    |     send(event_arrive)
    | end
    | % if skipFlag<-1e-6
    | %     send(event_skip)
    | % end
  function curVelVec_ = updateVelForTurn:
    | function curVelVec_ = updateVelForTurn()
    | dhead = turnHeadVel*Ts;
    | delevator = turnElvVel*Ts;
    | curVelVec_h = [curVelVec(1:2),0]';
    | tempCurVelVec = curVel*curVelVec_h/norm(curVelVec_h);
    | M_h = [...
    |      cos(dhead) sin(dhead) 0;
    |     -sin(dhead) cos(dhead) 0;
    |               0          0 1;];
    | M_e = [...
    |      cos(delevator) 0 -sin(delevator);
    |      0             1              0;
    |      sin(delevator) 0  cos(delevator);];          
    | temp = (M_e*M_h)'*tempCurVelVec;
    | curVelVec_ = temp';
  function [inPos,outPos] =calTurnInOutPos:
    | function [inPos,outPos] =calTurnInOutPos
    | inPos = curEndNav;
    | outPos = curEndNav;
    | if turnMode == 1
    |     inPos = curEndNav;
    |     outPos = curEndNav;
    | elseif turnMode == 2
    |     if ptIdx == numPts-1 % 当处于最后一段航线时
    |         inPos = curEndNav;
    |         outPos = -999*ones(size(path(ptIdx+1,1:3)));
    |     else
    |         nextNav = path(ptIdx+2,1:3);
    |         curVec = curEndNav-curStartNav;
    |         curVec(3) = 0; % 不考虑高度
    |         nextVec = nextNav-curEndNav;
    |         nextVec(3) = 0;
    |         lengthCurLine = norm(curVec);
    |         lengthNextLine = norm(nextVec);
    |         if lengthNextLine ~= 0
    |             %             if lengthCurLine<=dist || lengthNextLine<=dist
    |             %                 R = 1/2*min([lengthCurLine,lengthNextLine,dist]);
    |             %                 %             error('Turn radius is larger than the length of some path, which may cause unexpected results!');
    |             %             else
    |             %                 R = turnRadius;
    |             %             end
    |             R = turnRadius;
    |             angle1 = acos(dot([nextVec]/lengthNextLine,[curVec]/lengthCurLine));%asin(sum(cross([nextVec]/lengthNextLine,[curVec]/lengthCurLine)));
    |             angle_half = angle1/2;
    |             dist = R/abs(tan(pi/2-abs(angle_half)));
    |             while 1
    |                 if lengthCurLine<=dist || lengthNextLine<=dist
    |                     dist = 0.95*min(lengthCurLine,lengthNextLine);
    |                 else
    |                     break
    |                 end
    |             end
    |             inPos = curEndNav-curVec*dist/norm(curVec);
    |             outPos = curEndNav+nextVec*dist/norm(nextVec);
    |         else
    |             inPos = curEndNav;
    |             outPos = curEndNav;
    |         end
    |         if isnan(outPos)
    |             sl = 1;
    |         end
    |     end
    | end
    | if 0 % TEST
    |     figure;
    |     plot(curPos(1),curPos(2),'k+');hold on;
    |     plot(curEndNav(1),curEndNav(2),'ro');hold on;
    |     plot(curStartNav(1),curStartNav(2),'ro');hold on;
    |     plot(inPos(1),inPos(2),'bo');hold on;
    |     plot(outPos(1),outPos(2),'bo');hold on;
    |     plot(nextNav(1),nextNav(2),'ro');hold on;
    |     plot([curStartNav(1) curEndNav(1) nextNav(1)],[curStartNav(2) curEndNav(2) nextNav(2)],'r');hold on;
    |     axis equal
    |     grid on;
    | end
    | test = 1;
  function TESTFUNC:
    | function TESTFUNC
    | coder.extrinsic('fprintf')
    | % fprintf('\n');
    | % fprintf('head: %.2f\n',head*57.3);
    | % fprintf('headTurned: %.2f\n', head*57.3-head0*57.3);
    | % fprintf('head_flag: %d\n', abs(head-head0)>=headToTurn);
    | % fprintf('elevator_flag: %d\n', abs(elevator-elevator0)>=elevatorToTurn);
    | % fprintf('ptIdx: %d\n',ptIdx);
    | if isnan(curVelVec)
    |     sl = 1;
    | end
    | if isnan(sum(curPos))
    |     sl = 1;
    | end
    | % if isnan(headToTurn)
    | %     sl = 1;
    | % end
    | if ptIdx >=30
    |     sl = 1;
    | end
  function [path_,path_h_,path_v_] = calValidNavPts(initialpos,pathlist,finalpos):
    | function [path_,path_h_,path_v_] = calValidNavPts(initialpos,pathlist,finalpos)
    | %% 计算包括当前位置和额外指定终点在内的完整航路
    | % initialpos：进入导航模式时的单位所在位置
    | % pathlist：航路点序列
    | % finalpos:终点位置
    | %% 计算过程
    | path_ = [initialpos(1:3);pathlist(:,1:3);finalpos(1:3)]; % 形成完整航路数组
    | % path_最小点数为4（1起点+2航路+1终点），航路规划算法给出的pathlist中，
    | % 由[0,0,0]填充末尾不存在的位置点，因此在实际导航时，需将这些点去掉
    | for i = size(path_,1)-1:-1:4 
    |     if norm(path_(i,:)) == 0 % 处理末尾的[0,0,0],填充为终点位置坐标
    |         path_(i,:) = finalpos(1:3);
    |     else
    |         break;
    |     end
    | end
    | path_h_ = [path_(:,1:2) 0*path_(:,3)];
    | path_v_ = [0*path_(:,1) 0*path_(:,2) path_(:,3)];
    | test = 1; % 用于加断点的行
  function elevator_ = calElevatorForHeightManuv:
    | function elevator_ = calElevatorForHeightManuv
    | elevatorCmd = maxElevator;
    | dElevatorCmd = dElevator_cmd;
    | turnR = turnRadiusVertical;
    | premeter = 2*pi*turnR;
    | arcLength = premeter*2*elevatorCmd/2/pi;
    | tSpend = arcLength/curVel;
    | dist = turnR*tan(elevatorCmd);
    | turnH = dist*sin(elevatorCmd); 
    | 
    | targetHeight = path(ptIdx+1,3);
    | % startHeight = path(ptIdx,3);
    | startHeight = height0;
    | currentHeight = curPos(3);
    | restHeight = targetHeight-currentHeight;
    | passedHeight = currentHeight-startHeight;
    | absoluteErrHeight = targetHeight-startHeight;
    | if abs(absoluteErrHeight)>2*turnH 
    |     if elevator<=elevatorCmd && abs(passedHeight)<=turnH
    |         dElevator_ = sign(absoluteErrHeight)*dElevatorCmd;
    |         phase = 1;
    |     elseif abs(passedHeight)>abs(absoluteErrHeight)-turnH 
    |         dElevator_ = -sign(absoluteErrHeight)*dElevatorCmd;
    |         phase = 3;
    |     else
    |         dElevator_ = 0;
    |         phase = 2;
    |     end
    | else
    |     if abs(passedHeight)<1/2*abs(absoluteErrHeight)
    |         dElevator_ = sign(absoluteErrHeight)*dElevatorCmd;
    |         phase = 1;
    |     else
    |         dElevator_ = -sign(absoluteErrHeight)*dElevatorCmd;
    |         phase = 3;
    |     end
    | end
    | switch phase
    |     case 1
    |         elevator_ = elevator + dElevator_*Ts;
    |         if absoluteErrHeight>0
    |             elevator_ = min(elevator_,elevatorCmd);
    |         else
    |             elevator_ = max(elevator_,-elevatorCmd);
    |         end
    |     case 2
    |         elevator_ = sign(absoluteErrHeight)*elevatorCmd;
    |     case 3
    |         elevator_ = elevator + dElevator_*Ts;
    |         if absoluteErrHeight>0
    |             elevator_ = max(elevator_,0);
    |         else
    |             elevator_ = min(elevator_,0);
    |         end        
    |     otherwise
    |         elevator_ = 0;
    | end
  function [turnAngleVel_h,turnAngleVel_e,angleToTurn_h,angleToTurn_e] ...:
    | function [turnAngleVel_h,turnAngleVel_e,angleToTurn_h,angleToTurn_e] ...
    |     = calTurnPos()
    | nextNav = path(ptIdx+2,1:3);
    | curVec = curEndNav-curStartNav;
    | % curVec = curEndNav-curPos; 
    | curVec(3) = 0;
    | nextVec = nextNav-curEndNav;
    | nextVec(3) = 0;
    | lengthCurLine = norm(curVec);
    | lengthNextLine = norm(nextVec);
    | if lengthNextLine ~= 0 && lengthCurLine ~= 0
    |     angleToTurn_h_sym = asin(sum(cross(nextVec/lengthNextLine,curVec/lengthCurLine)));
    |     angleToTurn_h = acos(sum(dot(nextVec/lengthNextLine,curVec/lengthCurLine)));
    | else
    |     angleToTurn_h_sym = 0;
    |     angleToTurn_h = 0;
    | end
    | curElv = rem(atan2(curVec(3),curVec(2)),pi);
    | nextElv = rem(atan2(nextVec(3),nextVec(2)),pi);
    | if angleToTurn_h_sym >= 0
    |     flag_h = -1;  
    | else
    |     flag_h = 1;
    | end
    | perimeter = 2*pi*turnRadius;
    | timePerCircle = perimeter/curVel;
    | turnAngleVel_h = flag_h*2*pi/timePerCircle;%abs(angleToTurn_h)/timePerCircle;
    | turnAngleVel_e = (nextElv-curElv)/timePerCircle;
    | angleToTurn_h = abs(angleToTurn_h);
    | angleToTurn_e = nextElv-curElv;
    | if isnan(angleToTurn_h)
    |     sl = 1;
    | end

== matlab function myStateFlow/Navigator/Switch Case Action Subsystem2/For Each Subsystem/MATLAB Function ==
  data: u input; y output
function y = fcn(u)

y = u(:,:,1);

== matlab function myStateFlow/Navigator/Switch Case Action Subsystem2/For Each Subsystem/MATLAB Function1 ==
  data: u input; y output
function y = fcn(u)

y = u(1,:,1);

== matlab function myStateFlow/Navigator/Switch Case Action Subsystem2/For Each Subsystem/MATLAB Function2 ==
  data: u input; y output
function y = fcn(u)

y = u(1,:,1);

== matlab function myStateFlow/Navigator/Switch Case Action Subsystem2/For Each Subsystem/MATLAB Function3 ==
  data: u input; y output
function y = fcn(u)

y = u(1,:,1);

== matlab function myStateFlow/Navigator/Switch Case Action Subsystem2/For Each Subsystem/MATLAB Function4 ==
  data: u input; y output
function y = fcn(u)

y = u(1,:,1);

== matlab function myStateFlow/Navigator/Switch Case Action Subsystem2/For Each Subsystem/MATLAB Function5 ==
  data: u input; y output
function y = fcn(u)

y = u(1,:,1);

== matlab function myStateFlow/Navigator/Switch Case Action Subsystem2/MATLAB Function ==
  data: data input; dataout output; sizedata input
function dataout = fcn(data,sizedata)
dataout = zeros(size(sizedata));
dataout(1,:) = data;

== matlab function myStateFlow/Navigator/Switch Case Action Subsystem2/MATLAB Function1 ==
  data: data input; dataout output; sizedata input
function dataout = fcn(data,sizedata)
dataout = zeros(size(sizedata));
dataout(1,:) = data;
